simulink model "pendulo_pv_linear"  (R2020b)
settings: Solver=VariableStepAuto  StartTime=0.0  StopTime=100  FixedStep=1e-3  RelTol=1e-3
values from neighbouring files (symbols this model uses):
  controlador = projetarControlador(requisitos, planta)    [executarTudo.m]    (also in runAll.m; simular.m)
  planta = obterPlanta()    [codetest.m]    (also in executarTudo.m; nextState.m; runAll.m; simular.m)
  thetar = 0    [executarTudo.m]    (also in runAll.m)
undefined symbols (not defined in the file or in its folder): varCom, varMed
settings Model: Creator=davi  LastModifiedBy=alexandremaranhao
settings SolverCC: AlgebraicLoopSolver=LineSearch

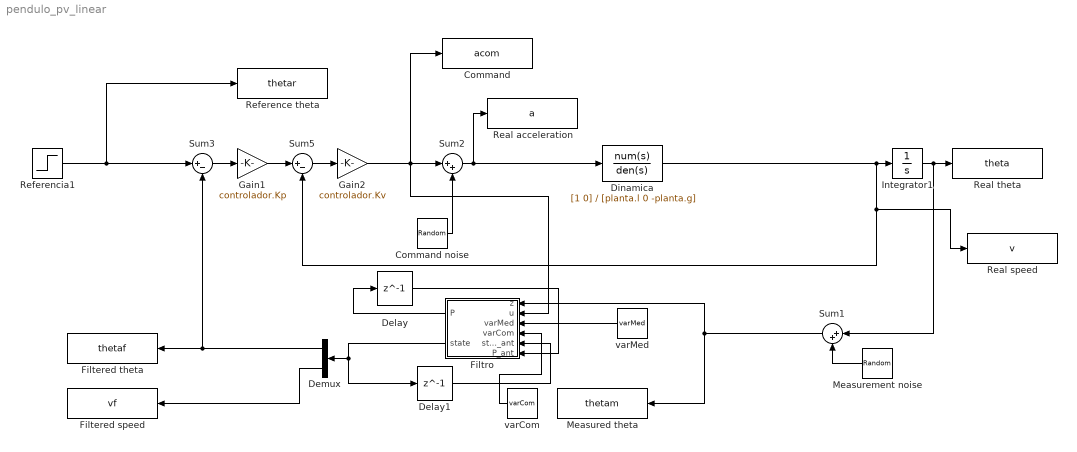
== system pendulo_pv_linear ==
  Command : ToWorkspace  VariableName=acom  SaveFormat=Structure With Time  SampleTime=-1
  Command noise : RandomNumber  Variance=varCom  SampleTime=1e-2
  Delay : Delay  DelayLength=1  InitialCondition=eye(2)  SampleTime=1e-2
  Delay1 : Delay  DelayLength=1  InitialCondition=[0;0]  SampleTime=1e-2
  Demux : Demux  Outputs=2
  Dinamica : TransferFcn  Numerator=[1 0]  Denominator=[planta.l 0 -planta.g]
  Filtered speed : ToWorkspace  VariableName=vf  SaveFormat=Structure With Time  SampleTime=-1
  Filtered theta : ToWorkspace  VariableName=thetaf  SaveFormat=Structure With Time  SampleTime=-1
  Filtro : MATLAB Function  TreatAsAtomicUnit=on  SystemSampleTime=1e-2
  Gain1 : Gain  Gain=controlador.Kp
  Gain2 : Gain  Gain=controlador.Kv
  Integrator1 : Integrator
  Measured theta : ToWorkspace  VariableName=thetam  SaveFormat=Structure With Time  SampleTime=-1
  Measurement noise : RandomNumber  Variance=varMed  SampleTime=1e-2
  Real acceleration : ToWorkspace  VariableName=a  SaveFormat=Structure With Time  SampleTime=-1
  Real speed : ToWorkspace  VariableName=v  SaveFormat=Structure With Time  SampleTime=-1
  Real theta : ToWorkspace  VariableName=theta  SaveFormat=Structure With Time  SampleTime=-1
  Reference theta : ToWorkspace  VariableName=thetar  SaveFormat=Structure With Time  SampleTime=-1
  Referencia1 : Step  Time=0  After=thetar  SampleTime=0
  Sum1 : Sum  Inputs=|++
  Sum2 : Sum  Inputs=|++
  Sum3 : Sum  Inputs=|+-
  Sum5 : Sum  Inputs=|+-
  varCom : Constant  Value=varCom
  varMed : Constant  Value=varMed
  wires:
  Measurement noise/1 -> Sum1/2
  Sum2/1 -> Dinamica/1, Real acceleration/1
  Command noise/1 -> Sum2/2
  Referencia1/1 -> Sum3/1, Reference theta/1
  Dinamica/1 -> Integrator1/1, Sum5/2, Real speed/1
  Integrator1/1 -> Real theta/1, Sum1/1
  Sum3/1 -> Gain1/1
  varMed/1 -> Filtro/3(varMed)
  varCom/1 -> Filtro/4(varCom)
  Sum1/1 -> Measured theta/1, Filtro/1(z)
  Filtro/2(state) -> Delay1/1, Demux/1
  Filtro/1(P) -> Delay/1
  Delay1/1 -> Filtro/5(state_ant)
  Delay/1 -> Filtro/6(P_ant)
  Demux/2 -> Filtered speed/1
  Demux/1 -> Sum3/2, Filtered theta/1
  Gain2/1 -> Filtro/2(u), Command/1, Sum2/1
  Gain1/1 -> Sum5/1
  Sum5/1 -> Gain2/1

== matlab function pendulo_pv_linear/Filtro ==
  settings: updateMethod=DISCRETE
  data: z input; u input; varMed input; varCom input; state_ant input; P_ant input; P output; state output
function [P, state] = fcn(z, u, varMed, varCom, state_ant, P_ant)

F = [1.0010    0.0100; 0.1963    1.0010];
G = [0.0001; 0.02];
n=2;
Q=G*varMed*G'; %covariance of process
R=varMed;        %covariance of measurement  

x_pred = F*state_ant + G*u;
P_pred = F*P_ant*F' + Q;

C = [1 0];
Kt = P_pred * C' * pinv(R + C*P_pred*C');
state = x_pred + Kt*(z-C*state_ant);
P = P_pred - Kt*C*P_pred;
% y = z;
end
